simulink model "main"  (R2021a)
settings: Solver=VariableStepAuto  StartTime=0.0  StopTime=5  RelTol=1e-3
libraries: aerolibutil x2, pid_lib x1
settings Model: Creator=l.ribeiro-lustosa  LastModifiedBy=l.ribeiro-lustosa

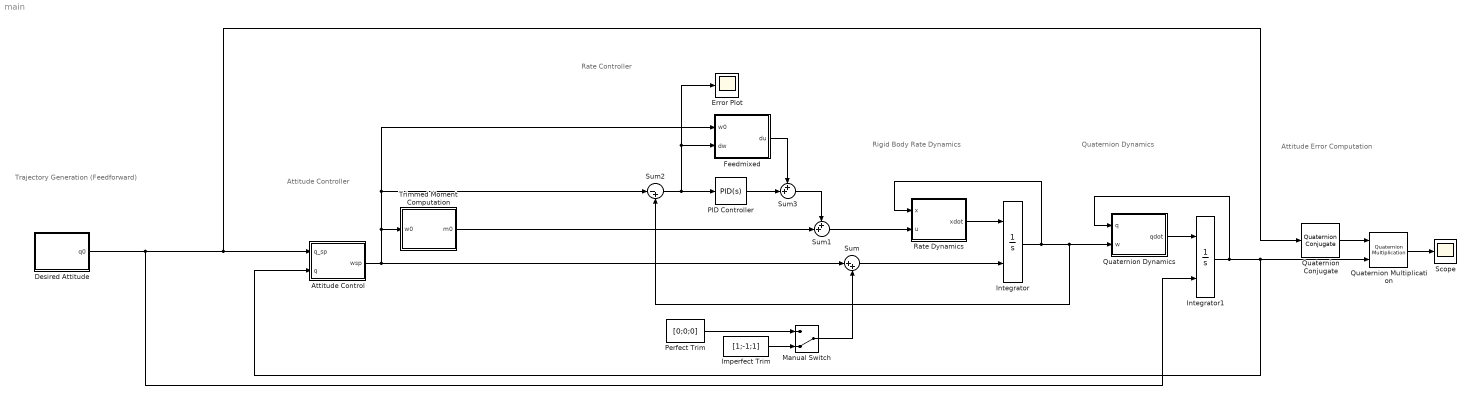
== system main ==
  note: Attitude Error Computation
  note: Attitude Controller
  note: Quaternion Dynamics
  note: Rate Controller
  note: Trajectory Generation (Feedforward)
  note: Rigid Body Rate Dynamics
  Attitude Control : MATLAB Function  TreatAsAtomicUnit=on
  Desired Attitude : MATLAB Function  TreatAsAtomicUnit=on
  Error Plot : Scope
  Feedmixed : MATLAB Function  TreatAsAtomicUnit=on
  Imperfect Trim : Constant  Value=[1;-1;1]
  Integrator : Integrator  InitialConditionSource=external
  Integrator1 : Integrator  InitialConditionSource=external
  Manual Switch : ManualSwitch  CurrentSetting=0
  PID Controller : pid_lib/PID Controller  Controller=PID  Form=Parallel  TimeDomain=Continuous-time  UseExternalTs=off  SampleTime=-1  IntegratorMethod=Forward Euler  FilterMethod=Forward Euler  ControllerParametersSource=internal  P=-10  I=-1  D=0  UseFilter=on  N=100  TunerSelectOption=Frequency Response Based  InitialConditionSource=internal  InitialConditionForIntegrator=0  InitialConditionForFilter=0  DifferentiatorICPrevScaledInput=0  ExternalReset=none  TrackingMode=off  Kt=1  LimitOutput=off  SatLimitsSource=internal  UpperSaturationLimit=inf  LowerSaturationLimit=-inf  LinearizeAsGain=on  AntiWindupMode=none  Kb=1  POutMin=[]  POutMax=[]  IOutMin=[]  IOutMax=[]  DOutMin=[]  DOutMax=[]  NOutMin=[]  NOutMax=[]  SumOutMin=[]  SumOutMax=[]  SaturationOutMin=[]  SaturationOutMax=[]  PParamMin=[]  PParamMax=[]  IParamMin=[]  IParamMax=[]  DParamMin=[]  DParamMax=[]  NParamMin=[]  NParamMax=[]  KbParamMin=[]  KbParamMax=[]  KtParamMin=[]  KtParamMax=[]  KbOutMin=[]  KbOutMax=[]  KtOutMin=[]  KtOutMax=[]  IntegratorOutMin=[]  IntegratorOutMax=[]  FilterOutMin=[]  FilterOutMax=[]  SumI1OutMin=[]  SumI1OutMax=[]  SumI2OutMin=[]  SumI2OutMax=[]  SumI3OutMin=[]  SumI3OutMax=[]  SumI4OutMin=[]  SumI4OutMax=[]  SumDOutMin=[]  SumDOutMax=[]  DifferentiatorOutMin=[]  DifferentiatorOutMax=[]  FilterDiffOutCoefMin=[]  FilterDiffOutCoefMax=[]  ReciprocalOutMin=[]  ReciprocalOutMax=[]  SumDenOutMin=[]  SumDenOutMax=[]  SumNumOutMin=[]  SumNumOutMax=[]  DivideOutMin=[]  DivideOutMax=[]  UdiffTsProdOutMin=[]  UdiffTsProdOutMax=[]  NTsProdOutMin=[]  NTsProdOutMax=[]  UintegralTsProdOutMin=[]  UintegralTsProdOutMax=[]  UngainTsProdOutMin=[]  UngainTsProdOutMax=[]  IntegratorContinuousStateAttributes=''  IntegratorStateMustResolveToSignalObject=off  IntegratorRTWStateStorageClass=Auto  FilterContinuousStateAttributes=''  FilterStateMustResolveToSignalObject=off  FilterRTWStateStorageClass=Auto  ParallelPVariant=InternalParameters  IdealPVariant=Disabled  IVariant=InternalParameters  DVariant=InternalParameters  IntegratorVariant=Continuous  SatVariant=Disabled  AWVariant=Passthrough  PCopyVariant=Disabled  TRVariant=Disabled  FdbkBlocksVariant=Forward  IdealPFdbkVariant=Disabled  SatFdbkVariant=Disabled  DerivativeFilterVariant=ContFilter  NVariant=InternalParameters  NCopyVariant=Disabled  FilterICVariant=InternalICsFilter  IntegratorICVariant=InternalICs  ExternalResetVariant=Disabled  TRSumVariant=Passthrough  SumFdbkVariant=Disabled  SumVariant=Sum_PID  TsampFilterVariant=InternalTs  TsampNgainVariant=Passthrough  TsampIntegralVariant=Passthrough  ExternalSaturationOutDataTypeStr=Inherit: Same as second input
  Perfect Trim : Constant  Value=[0;0;0]
  Quaternion Conjugate : aerolibutil/Quaternion Conjugate
      settings: SourceProductBaseCode=AE
  Quaternion Multiplication : aerolibutil/Quaternion Multiplication
  Quaternion Dynamics : MATLAB Function  TreatAsAtomicUnit=on
  Rate Dynamics : MATLAB Function  TreatAsAtomicUnit=on
  Scope : Scope
  Sum : Sum  Inputs=|++
  Sum1 : Sum  Inputs=++|
  Sum2 : Sum  Inputs=|-+
  Sum3 : Sum  Inputs=++|
  Trimmed Moment Computation : MATLAB Function  TreatAsAtomicUnit=on
  wires:
  Rate Dynamics/1(xdot) -> Integrator/1
  Integrator/1 -> Quaternion Dynamics/2(w), Sum2/2, Rate Dynamics/1(x)
  Sum/1 -> Integrator/2
  Perfect Trim/1 -> Manual Switch/1
  Imperfect Trim/1 -> Manual Switch/2
  Manual Switch/1 -> Sum/2
  Sum1/1 -> Rate Dynamics/2(u)
  Sum2/1 -> Error Plot/1, Feedmixed/2(dw), PID Controller/1
  Sum3/1 -> Sum1/1
  PID Controller/1 -> Sum3/2
  Quaternion Dynamics/1(qdot) -> Integrator1/1
  Integrator1/1 -> Quaternion Dynamics/1(q), Attitude Control/2(q), Quaternion Multiplication/2
  Attitude Control/1(wsp) -> Sum2/1, Feedmixed/1(w0), Trimmed Moment Computation/1(w0), Sum/1
  Desired Attitude/1(q0) -> Integrator1/2, Quaternion Conjugate/1, Attitude Control/1(q_sp)
  Trimmed Moment Computation/1(m0) -> Sum1/2
  Feedmixed/1(du) -> Sum3/1
  Quaternion Conjugate/1 -> Quaternion Multiplication/1
  Quaternion Multiplication/1 -> Scope/1

== matlab function main/Trimmed Moment Computation ==
  data: w0 input; m0 output; J parameter
function m0 = fcn(w0,J)

m0 = cross(w0,J*w0);

== matlab function main/Rate Dynamics ==
  data: x input; u input; xdot output; J parameter
function xdot = fcn(x,u,J)

%% Newton's Second Law for Rotation
xdot = J\( u - cross(x,J*x) );

== matlab function main/Desired Attitude ==
  data: q0 output
function q0 = fcn()

q0 = [1;2;3;4];
q0 = q0/norm(q0);

== matlab function main/Feedmixed ==
  data: w0 input; dw input; du output; J parameter
function du = fcn(w0,dw,J)

%% model-based mixed feedback + feedforward term
du = cross( w0, J*dw );

== matlab function main/Attitude Control ==
  data: q_sp input; q input; wsp output
function wsp = fcn(q_sp,q)
%MC_ATT_CONTROL Summary of this function goes here
%   Missing saturation!!! Implement it later!!!
% x = (EMPTY) : 
% u = (q_sp, q, yawspeed_setpoint) in R^(9x1)
% y = (rate_sp) in R⁽3x1)

% these are the *default* params obtained in the doc:
% https://docs.px4.io/master/en/advanced_config/parameter_reference.html
YAW_W = 0.4;    
PROPORTIONAL_GAIN = [6.5;6.5;2.8];

yawspeed_setpoint = 0;

% calculate reduced desired attitude neglecting vehicle's yaw to prioritize roll and pitch
e_z = quat2dcm(q')'*[0;0;1];
e_z_d = quat2dcm(q_sp')'*[0;0;1];
qd_red = quat_red(e_z,e_z_d);

if (abs(qd_red(2)) > (1.0 - 1e-5) || abs(qd_red(3)) > (1.0 - 1e-5))
		% In the infinitesimal corner case where the vehicle and thrust have the completely opposite direction,
		% full attitude control anyways generates no yaw input and directly takes the combination of
		% roll and pitch leading to the correct desired yaw. Ignoring this case would still be totally safe and stable.
		qd_red = q_sp;
else
		% transform rotation from current to desired thrust vector into a world frame reduced desired attitude
		qd_red = quatmultiply(qd_red',q')';
end

% mix full and reduced desired attitude
q_mix = quatmultiply( quatinv(qd_red'), q_sp')';
q_mix =	canonicalize(q_mix);
% catch numerical problems with the domain of acosf and asinf
if (q_mix(1)>1)
    q_mix(1) = 1;
elseif (q_mix(1)<-1)
    q_mix(1) = -1;
end
if (q_mix(4)>1)
    q_mix(4) = 1;
elseif (q_mix(4)<-1)
    q_mix(4) = -1;
end

q_sp = quatmultiply(qd_red',[cos(YAW_W * acos(q_mix(1))); 0; 0; sin(YAW_W * asin(q_mix(4)))]')';

% quaternion attitude control law, qe is rotation from q to qd
qe = quatmultiply(quatinv(q'),q_sp')';

% using sin(alpha/2) scaled rotation axis as attitude error (see quaternion definition by axis angle)
% also taking care of the antipodal unit quaternion ambiguity
qec = canonicalize(qe);
eq = 2.0 * qec(2:4,1);

% calculate angular rates setpoint
rate_sp = eq.*PROPORTIONAL_GAIN;

% Feed forward the yaw setpoint rate.
% yawspeed_setpoint is the feed forward commanded rotation around the world z-axis,
% but we need to apply it in the body frame (because _rates_sp is expressed in the body frame).
% Therefore we infer the world z-axis (expressed in the body frame) by taking the last column of R.transposed (== q.inversed)
% and multiply it by the yaw setpoint rate (yawspeed_setpoint).
% This yields a vector representing the commanded rotatation around the world z-axis expressed in the body frame
% such that it can be added to the rates setpoint.
rate_sp = rate_sp + quat2dcm(quatinv(q'))*[1;0;0] * yawspeed_setpoint;

wsp = rate_sp;

end

% Quaternion from two vectors
% Generates shortest rotation from source to destination vector
%
% @param dst destination vector (no need to normalize)
% @param src source vector (no need to normalize)
% @param eps epsilon threshold which decides if a value is considered zero
%
function q = quat_red(src, dst)

q = zeros(4,1); % mem alloc
eps = 1e-5;

cr = cross(src,dst);
dt = dot(src,dst);

if (norm(cr) < eps && dt < 0)
    % handle corner cases with 180 degree rotations
    % if the two vectors are parallel, cross product is zero
    % if they point opposite, the dot product is negative
    cr = abs(src);
    if (cr(1) < cr(2))
        if (cr(1) < cr(3))
            cr = [1;0;0];
        else
            cr = [0;0;1];
        end
    else
        if (cr(2) < cr(3))
            cr = [0;1;0];
        else
            cr = [0;0;1];
        end
    end
    q(1) = 0;
    cr = cross(src,cr);
else
    % normal case, do half-way quaternion solution
    q(1) = dt + norm(src)*norm(dst);
end

q(2) = cr(1);
q(3) = cr(2);
q(4) = cr(3);
q = q/norm(q);

end

%
% Return canonical form of the quaternion
%
% @return quaternion in canonical form
function q = canonicalize(qi)

FLT_EPSILON = 1.19209e-07;

q = qi;

for i=1:4
    if (abs(q(i)) > FLT_EPSILON)
        q = q * sign(q(i));
        break;
    end
end

end

function dcm = quat2dcm( q )
%  QUAT2DCM Convert quaternion to direction cosine matrix.
%   N = QUAT2DCM( Q ) calculates the direction cosine matrix, N, for a
%   given quaternion, Q.  Input Q is an M-by-4 matrix containing M
%   quaternions.  N returns a 3-by-3-by-M matrix of direction cosine 
%   matrices.  The direction cosine matrix performs the coordinate
%   transformation of a vector in inertial axes to a vector in body axes.
%   Each element of Q must be a real number.  Additionally, Q has its
%   scalar number as the first column. 
%
%   Examples:
%
%   Determine the direction cosine matrix from q = [1 0 1 0]:
%      dcm = quat2dcm([1 0 1 0])
%
%   Determine the direction cosine matrices from multiple quaternions:
%      q = [1 0 1 0; 1 0.5 0.3 0.1];
%      dcm = quat2dcm(q)
%
%   See also ANGLE2DCM, DCM2ANGLE, DCM2QUAT, ANGLE2QUAT, QUAT2ANGLE, QUATROTATE. 

%   Copyright 2000-2007 The MathWorks, Inc.

qin = quatnormalize( q );

dcm = zeros(3,3,size(qin,1));

dcm(1,1,:) = qin(:,1).^2 + qin(:,2).^2 - qin(:,3).^2 - qin(:,4).^2;
dcm(1,2,:) = 2.*(qin(:,2).*qin(:,3) + qin(:,1).*qin(:,4));
dcm(1,3,:) = 2.*(qin(:,2).*qin(:,4) - qin(:,1).*qin(:,3));
dcm(2,1,:) = 2.*(qin(:,2).*qin(:,3) - qin(:,1).*qin(:,4));
dcm(2,2,:) = qin(:,1).^2 - qin(:,2).^2 + qin(:,3).^2 - qin(:,4).^2;
dcm(2,3,:) = 2.*(qin(:,3).*qin(:,4) + qin(:,1).*qin(:,2));
dcm(3,1,:) = 2.*(qin(:,2).*qin(:,4) + qin(:,1).*qin(:,3));
dcm(3,2,:) = 2.*(qin(:,3).*qin(:,4) - qin(:,1).*qin(:,2));
dcm(3,3,:) = qin(:,1).^2 - qin(:,2).^2 - qin(:,3).^2 + qin(:,4).^2;

end

== matlab function main/Quaternion Dynamics ==
  data: q input; w input; qdot output
function qdot = fcn(q,w)

%% Quaternion kinematics
Omega = [0 -w(3) w(2); w(3) 0 -w(1); -w(2) w(1) 0];
qdot = 1/2*[0 -w'; w -Omega]*q;
